simulink library "tpm"  (R2021b)
settings: Solver=VariableStepAuto  StartTime=0.0  StopTime=10.0  RelTol=1e-3
undefined symbols (not defined in the file or in its folder): ENUM_AN_LF, ENUM_AN_LR, ENUM_AN_RF, ENUM_AN_RR, ENUM_POWERSTA_OFF, ENUM_POWERSTA_OFFA, ENUM_POWERSTA_OFFC, ENUM_POWERSTA_ON, ENUM_POWERSTA_READY, ENUM_POWERSTA_STANDBY, ENUM_PWRSTASW_OFF, ENUM_PWRSTASW_OFFA, ENUM_PWRSTASW_OFFCHVCHRG, ENUM_PWRSTASW_STANDBY, ENUM_TPMSSNESORIDREGSTA_START, FALSE, KTPM_DataInVehSpdThreshold_kph, KTPM_Delay_raw8, KTPM_DiagLearn_flg, KTPM_TPMSModelVersion_raw, KTPM_WhlRotDir_enum_ovrdflg, KTPM_WhlRotDir_enum_ovrdval, TRUE, ZERO_FLOAT, ZERO_INT
libraries: simulink x58, $bdroot x27, hcu_lib x24
(part 7 of 9)

== system tpm/TPM/TPMS/TPMS/Learn/AutoLocation/IDIdentify/Subsystem7/Enabled Subsystem1 ==
  C : Inport
  LFM1 : Inport  Port=2
  Enable : EnablePort
  Data Type Conversion{1..8} (8 alike) : DataTypeConversion  OutDataTypeStr=int16
  Data Type Conversion9 : DataTypeConversion  OutDataTypeStr=uint8
  MATLAB Function : MATLAB Function  TreatAsAtomicUnit=on
  Unit Delay{1..8} (8 alike) : UnitDelay  SampleTime=-1  HasFrameUpgradeWarning=on
  S : Outport
  wires:
  [X9] -> MATLAB Function/10(X9)
  Unit Delay8/1 -> Data Type Conversion8/1
  Data Type Conversion8/1 -> [X9]
  MATLAB Function/9(Y9) -> Unit Delay8/1
  MATLAB Function/8(Y8) -> Unit Delay7/1
  Data Type Conversion7/1 -> [X8]
  Unit Delay7/1 -> Data Type Conversion7/1
  Unit Delay4/1 -> Data Type Conversion6/1
  MATLAB Function/7(Y7) -> Unit Delay4/1
  Data Type Conversion6/1 -> [X7]
  [X8] -> MATLAB Function/9(X8)
  [X7] -> MATLAB Function/8(X7)
  [X6] -> MATLAB Function/7(X6)
  [X5] -> MATLAB Function/6(X5)
  Data Type Conversion5/1 -> [X6]
  Data Type Conversion4/1 -> [X5]
  MATLAB Function/5(Y5) -> Unit Delay5/1
  MATLAB Function/6(Y6) -> Unit Delay6/1
  Unit Delay5/1 -> Data Type Conversion4/1
  Unit Delay6/1 -> Data Type Conversion5/1
  [X4] -> MATLAB Function/5(X4)
  [X3] -> MATLAB Function/4(X3)
  [X2] -> MATLAB Function/3(X2)
  Unit Delay3/1 -> Data Type Conversion3/1
  Unit Delay2/1 -> Data Type Conversion2/1
  Unit Delay1/1 -> Data Type Conversion1/1
  MATLAB Function/4(Y4) -> Unit Delay3/1
  MATLAB Function/3(Y3) -> Unit Delay2/1
  MATLAB Function/2(Y2) -> Unit Delay1/1
  C/1 -> MATLAB Function/1(C)
  MATLAB Function/1(S) -> Data Type Conversion9/1
  LFM1/1 -> MATLAB Function/2(Min)
  Data Type Conversion1/1 -> [X2]
  Data Type Conversion2/1 -> [X3]
  Data Type Conversion3/1 -> [X4]
  Data Type Conversion9/1 -> S/1

== system tpm/TPM/TPMS/TPMS/Learn/AutoLocation/IDIdentify/Subsystem7/Enabled Subsystem2 ==
  C : Inport
  LFM1 : Inport  Port=2
  Enable : EnablePort
  Data Type Conversion{1..8} (8 alike) : DataTypeConversion  OutDataTypeStr=int16
  Data Type Conversion9 : DataTypeConversion  OutDataTypeStr=uint8
  MATLAB Function : MATLAB Function  TreatAsAtomicUnit=on
  Unit Delay{1..8} (8 alike) : UnitDelay  SampleTime=-1  HasFrameUpgradeWarning=on
  S : Outport
  wires:
  Data Type Conversion3/1 -> [X4]
  Data Type Conversion2/1 -> [X3]
  Data Type Conversion1/1 -> [X2]
  LFM1/1 -> MATLAB Function/2(Min)
  MATLAB Function/1(S) -> Data Type Conversion9/1
  C/1 -> MATLAB Function/1(C)
  MATLAB Function/2(Y2) -> Unit Delay1/1
  MATLAB Function/3(Y3) -> Unit Delay2/1
  MATLAB Function/4(Y4) -> Unit Delay3/1
  Unit Delay1/1 -> Data Type Conversion1/1
  Unit Delay2/1 -> Data Type Conversion2/1
  Unit Delay3/1 -> Data Type Conversion3/1
  [X2] -> MATLAB Function/3(X2)
  [X3] -> MATLAB Function/4(X3)
  [X4] -> MATLAB Function/5(X4)
  Unit Delay6/1 -> Data Type Conversion5/1
  Unit Delay5/1 -> Data Type Conversion4/1
  MATLAB Function/6(Y6) -> Unit Delay6/1
  MATLAB Function/5(Y5) -> Unit Delay5/1
  Data Type Conversion4/1 -> [X5]
  Data Type Conversion5/1 -> [X6]
  [X5] -> MATLAB Function/6(X5)
  [X6] -> MATLAB Function/7(X6)
  [X7] -> MATLAB Function/8(X7)
  [X8] -> MATLAB Function/9(X8)
  Data Type Conversion6/1 -> [X7]
  MATLAB Function/7(Y7) -> Unit Delay4/1
  Unit Delay4/1 -> Data Type Conversion6/1
  Unit Delay7/1 -> Data Type Conversion7/1
  Data Type Conversion7/1 -> [X8]
  MATLAB Function/8(Y8) -> Unit Delay7/1
  MATLAB Function/9(Y9) -> Unit Delay8/1
  Data Type Conversion8/1 -> [X9]
  Unit Delay8/1 -> Data Type Conversion8/1
  [X9] -> MATLAB Function/10(X9)
  Data Type Conversion9/1 -> S/1

== system tpm/TPM/TPMS/TPMS/Learn/AutoLocation/IDIdentify/Subsystem7/Enabled Subsystem3 ==
  C : Inport
  LFM1 : Inport  Port=2
  Enable : EnablePort
  Data Type Conversion{1..8} (8 alike) : DataTypeConversion  OutDataTypeStr=int16
  Data Type Conversion9 : DataTypeConversion  OutDataTypeStr=uint8
  MATLAB Function : MATLAB Function  TreatAsAtomicUnit=on
  Unit Delay{1..8} (8 alike) : UnitDelay  SampleTime=-1  HasFrameUpgradeWarning=on
  S : Outport
  wires:
  [X9] -> MATLAB Function/10(X9)
  Unit Delay8/1 -> Data Type Conversion8/1
  Data Type Conversion8/1 -> [X9]
  MATLAB Function/9(Y9) -> Unit Delay8/1
  MATLAB Function/8(Y8) -> Unit Delay7/1
  Data Type Conversion7/1 -> [X8]
  Unit Delay7/1 -> Data Type Conversion7/1
  Unit Delay4/1 -> Data Type Conversion6/1
  MATLAB Function/7(Y7) -> Unit Delay4/1
  Data Type Conversion6/1 -> [X7]
  [X8] -> MATLAB Function/9(X8)
  [X7] -> MATLAB Function/8(X7)
  [X6] -> MATLAB Function/7(X6)
  [X5] -> MATLAB Function/6(X5)
  Data Type Conversion5/1 -> [X6]
  Data Type Conversion4/1 -> [X5]
  MATLAB Function/5(Y5) -> Unit Delay5/1
  MATLAB Function/6(Y6) -> Unit Delay6/1
  Unit Delay5/1 -> Data Type Conversion4/1
  Unit Delay6/1 -> Data Type Conversion5/1
  [X4] -> MATLAB Function/5(X4)
  [X3] -> MATLAB Function/4(X3)
  [X2] -> MATLAB Function/3(X2)
  Unit Delay3/1 -> Data Type Conversion3/1
  Unit Delay2/1 -> Data Type Conversion2/1
  Unit Delay1/1 -> Data Type Conversion1/1
  MATLAB Function/4(Y4) -> Unit Delay3/1
  MATLAB Function/3(Y3) -> Unit Delay2/1
  MATLAB Function/2(Y2) -> Unit Delay1/1
  C/1 -> MATLAB Function/1(C)
  MATLAB Function/1(S) -> Data Type Conversion9/1
  LFM1/1 -> MATLAB Function/2(Min)
  Data Type Conversion1/1 -> [X2]
  Data Type Conversion2/1 -> [X3]
  Data Type Conversion3/1 -> [X4]
  Data Type Conversion9/1 -> S/1

== system tpm/TPM/TPMS/TPMS/Learn/AutoLocation/IDIdentify/Subsystem7/Enabled Subsystem5 ==
  C : Inport
  LFM1 : Inport  Port=2
  Enable : EnablePort
  Data Type Conversion{1..8} (8 alike) : DataTypeConversion  OutDataTypeStr=int16
  Data Type Conversion9 : DataTypeConversion  OutDataTypeStr=uint8
  MATLAB Function : MATLAB Function  TreatAsAtomicUnit=on
  Unit Delay{1..8} (8 alike) : UnitDelay  SampleTime=-1  HasFrameUpgradeWarning=on
  S : Outport
  wires:
  Data Type Conversion3/1 -> [X4]
  Data Type Conversion2/1 -> [X3]
  Data Type Conversion1/1 -> [X2]
  LFM1/1 -> MATLAB Function/2(Min)
  MATLAB Function/1(S) -> Data Type Conversion9/1
  C/1 -> MATLAB Function/1(C)
  MATLAB Function/2(Y2) -> Unit Delay1/1
  MATLAB Function/3(Y3) -> Unit Delay2/1
  MATLAB Function/4(Y4) -> Unit Delay3/1
  Unit Delay1/1 -> Data Type Conversion1/1
  Unit Delay2/1 -> Data Type Conversion2/1
  Unit Delay3/1 -> Data Type Conversion3/1
  [X2] -> MATLAB Function/3(X2)
  [X3] -> MATLAB Function/4(X3)
  [X4] -> MATLAB Function/5(X4)
  Unit Delay6/1 -> Data Type Conversion5/1
  Unit Delay5/1 -> Data Type Conversion4/1
  MATLAB Function/6(Y6) -> Unit Delay6/1
  MATLAB Function/5(Y5) -> Unit Delay5/1
  Data Type Conversion4/1 -> [X5]
  Data Type Conversion5/1 -> [X6]
  [X5] -> MATLAB Function/6(X5)
  [X6] -> MATLAB Function/7(X6)
  [X7] -> MATLAB Function/8(X7)
  [X8] -> MATLAB Function/9(X8)
  Data Type Conversion6/1 -> [X7]
  MATLAB Function/7(Y7) -> Unit Delay4/1
  Unit Delay4/1 -> Data Type Conversion6/1
  Unit Delay7/1 -> Data Type Conversion7/1
  Data Type Conversion7/1 -> [X8]
  MATLAB Function/8(Y8) -> Unit Delay7/1
  MATLAB Function/9(Y9) -> Unit Delay8/1
  Data Type Conversion8/1 -> [X9]
  Unit Delay8/1 -> Data Type Conversion8/1
  [X9] -> MATLAB Function/10(X9)
  Data Type Conversion9/1 -> S/1

== system tpm/TPM/TPMS/TPMS/Learn/AutoLocation/WheelPosition/Subsystem/delay0 ==
  In1 : Inport
  Action Port : ActionPort
  Delay5 : Delay  DelayLength=0
  Out1 : Outport
  wires:
  In1/1 -> Delay5/1
  Delay5/1 -> Out1/1

== system tpm/TPM/TPMS/TPMS/Learn/AutoLocation/WheelPosition/Subsystem/delay1 ==
  In1 : Inport
  Action Port : ActionPort
  Delay5 : Delay  DelayLength=1
  Out1 : Outport
  wires:
  In1/1 -> Delay5/1
  Delay5/1 -> Out1/1

== system tpm/TPM/TPMS/TPMS/Learn/AutoLocation/WheelPosition/Subsystem/delay2 ==
  In1 : Inport
  Action Port : ActionPort
  Delay5 : Delay
  Out1 : Outport
  wires:
  In1/1 -> Delay5/1
  Delay5/1 -> Out1/1

== system tpm/TPM/TPMS/TPMS/Learn/AutoLocation/WheelPosition/Subsystem/delay3 ==
  In1 : Inport
  Action Port : ActionPort
  Delay5 : Delay  DelayLength=3
  Out1 : Outport
  wires:
  In1/1 -> Delay5/1
  Delay5/1 -> Out1/1

== system tpm/TPM/TPMS/TPMS/Learn/AutoLocation/WheelPosition/Subsystem/delay4 ==
  In1 : Inport
  Action Port : ActionPort
  Delay5 : Delay  DelayLength=4
  Out1 : Outport
  wires:
  Delay5/1 -> Out1/1
  In1/1 -> Delay5/1

== system tpm/TPM/TPMS/TPMS/Learn/AutoLocation/WheelPosition/Subsystem/delay5 ==
  In1 : Inport
  Action Port : ActionPort
  Delay5 : Delay  DelayLength=5
  Out1 : Outport
  wires:
  In1/1 -> Delay5/1
  Delay5/1 -> Out1/1

== system tpm/TPM/TPMS/TPMS/Learn/AutoLocation/WheelPosition/Subsystem/delay6 ==
  In1 : Inport
  Action Port : ActionPort
  Delay5 : Delay  DelayLength=6
  Out1 : Outport
  wires:
  Delay5/1 -> Out1/1
  In1/1 -> Delay5/1

== system tpm/TPM/TPMS/TPMS/Learn/AutoLocation/WheelPosition/Subsystem/delay7 ==
  In1 : Inport
  Action Port : ActionPort
  Delay5 : Delay  DelayLength=7
  Out1 : Outport
  wires:
  In1/1 -> Delay5/1
  Delay5/1 -> Out1/1

== system tpm/TPM/TPMS/TPMS/Learn/AutoLocation/WheelPosition/Subsystem/delay8 ==
  In1 : Inport
  Action Port : ActionPort
  Delay5 : Delay  DelayLength=8
  Out1 : Outport
  wires:
  Delay5/1 -> Out1/1
  In1/1 -> Delay5/1

== matlab function tpm/TPM/TPMS/TPMS/Learn/AutoLocation/IDIdentify/Subsystem7/Enabled Subsystem5/MATLAB Function ==
  data: C input; S output; Min input; X2 input; X3 input; X4 input; Y2 output; Y3 output; Y4 output; X5 input; X6 input; X7 input; X8 input; X9 input; Y5 output; Y6 output; Y7 output; Y8 output; Y9 output
function [S,Y2,Y3,Y4,Y5,Y6,Y7,Y8,Y9]   = fcn(C,Min,X2,X3,X4,X5,X6,X7,X8,X9)
Y=int16([X2 X3 X4 X5 X6 X7 X8 X9 Min]);
if (C<9)
    S=300;
else
    B=sort(Y);
    D=zeros(1,length(B));
    for i=1:1:length(D)
        if (i~=length(D))
            D(i)=B(i+1)-B(i);
        else
            if (B(length(D))-B(1)>B(1)+96-B(length(D)))
                D(length(D))=B(1)+96-B(length(D));
            else
                D(length(D))=B(length(D))-B(1);
            end
        end
    end

    [K,I]=sort(D);
    S=sum(K(1:7));
end
Y2=Y(2);
Y3=Y(3);
Y4=Y(4);
Y5=Y(5);
Y6=Y(6);
Y7=Y(7);
Y8=Y(8);
Y9=Y(9);

== stateflow chart tpm/TPM/TPMS/TPMS/Learn/AutoLocation/WheelPosition/Chart2 ==
  state Start
    state Forward
      en:
      a=(VTPM_RFWpos_raw+Delta);
      b=(VTPM_RFWpos_raw+Delta)/96;
      VTPM_RFWpos_raw=a-b*96;
    state Else
    state Backward
      en:
      a=(VTPM_RFWpos_raw+Delta);
      b=(VTPM_RFWpos_raw+Delta)/96;
      VTPM_RFWpos_raw=a-b*96;
    (default) -> (junction 54) : {VTPM_RFWpos_raw=0; Delta=0; PulseCountBuf=VINP_RFPulseCount_cnt;}
    Start -> (junction 54) : [hasChanged(VINP_RFPulseCount_cnt)]....
        | {Delta=VINP_RFPulseCount_cnt-PulseCountBuf;
        | PulseCountBuf=VINP_RFPulseCount_cnt;}
    (junction 54) -> (junction 47) [order 1] : [VPMM_PowerSta_enum!=ENUM_PWRSTASW_OFF&&....
        |  VPMM_PowerSta_enum!=ENUM_PWRSTASW_OFFCHVCHRG&&...
        |  VPMM_PowerSta_enum!=ENUM_PWRSTASW_OFFA&&....
        |  VPMM_PowerSta_enum!=ENUM_PWRSTASW_STANDBY&&....
        |  VINP_RFPulseCountV_flg==false]
    (junction 47) -> (junction 6) [order 1] : [VTPM_RFWhlRotDir_enum==1]
    (junction 6) -> Forward [order 1] : [Delta>0]
    (junction 54) -> Else [order 2]
    (junction 47) -> (junction 48) [order 2]
    (junction 6) -> (junction 10) [order 2] : [Delta<0]
    (junction 10) -> Forward : {Delta=Delta+256;}
    (junction 48) -> Else [order 2]
    (junction 48) -> (junction 14) [order 1] : [VTPM_RFWhlRotDir_enum==2]
    (junction 14) -> Backward [order 1] : [Delta>0]{Delta=-Delta+96;}
    (junction 14) -> (junction 16) [order 2] : [Delta<0]
    (junction 16) -> Backward : {Delta=-Delta+128;}
  data: VPMM_PowerSta_enum input; VINP_RFPulseCount_cnt input; VINP_RFPulseCountV_flg input; VTPM_RFWhlRotDir_enum input; VTPM_RFWpos_raw output int16; a local int16; b local int16; Delta local int16; PulseCountBuf local int16; ENUM_PWRSTASW_OFF parameter; ENUM_PWRSTASW_OFFA parameter; ENUM_PWRSTASW_OFFCHVCHRG parameter; ENUM_PWRSTASW_STANDBY parameter

== stateflow chart tpm/TPM/TPMS/TPMS/Learn/AutoLocation/IDIdentify/unlearnsensorfail /Chart ==
  state FLSAH
    en:
    VTPM_unlearnSfali_flg=VINP_FlashunlearnSfali_flg;
  state VINP_TPMSResButt_flg
    en:
    VTPM_unlearnSfali_flg=false;
    VTPM_GSX_flg=false;
    VTPM_Idunlock_cnt=0;
    VTPM_GSS1_cnt=0;
    VTPM_GSS2_cnt=0;
    VTPM_GSS3_cnt=0;
    VTPM_GSS4_cnt=0;
    VTPM_Idunlockkeep_cnt=0;
    VTPM_unlockpopup_flg=false;
  state ALfin
    en:
    VTPM_GSX_flg=false;
    VTPM_unlearnSfali_flg=false;
    VTPM_unlockpopup_flg=false;
  state vehspeedthreshold
    en:
    VTPM_Idunlock_cnt=0;
    VTPM_GSS1_cnt=0;
    VTPM_GSS2_cnt=0;
    VTPM_GSS3_cnt=0;
    VTPM_GSS4_cnt=0;
  state locationdone
    en:
    VTPM_GSX_flg=false;
    VTPM_unlearnSfali_flg=false;
    VTPM_unlockpopup_flg=false;
  state unlearnsensorfail
    (default) -> (junction 83) : {VTPM_Idunlock_cnt=0;
        | VTPM_GSS1_cnt=0;
        | VTPM_GSS2_cnt=0;
        | VTPM_GSS3_cnt=0;
        | VTPM_GSS4_cnt=0;
        | }
    unlearnsensorfail -> (junction 83) [order 1] : [!VTPM_IDLOCK_flg]
    (junction 83) -> (junction 86) [order 1] : [VTPM_IDLOCK_flg]
    (junction 83) -> (junction 211) [order 2] : {VTPM_Idunlock_cnt+=1;
        | VTPM_Idunlockkeep_cnt+=1;}
    (junction 86) -> (junction 90) : {VTPM_unlockpopup_flg=false;}
    (junction 211) -> (junction 212) [order 1] : [VTPM_Idunlockkeep_cnt==30000||VTPM_unlockpopup_flg==true]
    (junction 211) -> (junction 215) [order 2]
    (junction 212) -> (junction 88) : {VTPM_unlockpopup_flg=true;}
    (junction 88) -> (junction 103) [order 1] : [VTPM_Idunlock_cnt==48000||VTPM_unlearnSfali_flg==true]
    (junction 88) -> (junction 105) [order 2]
    (junction 103) -> (junction 107) : {VTPM_unlearnSfali_flg=true;}
    unlearnsensorfail -> (junction 90) [order 2] : [VTPM_GSX_flg==true||VTPM_IDLOCK_flg]{VTPM_unlockpopup_flg=false;}
    (junction 90) -> (junction 132) [order 1] : [VTPM_GS1_flg==true]
    (junction 90) -> (junction 144) [order 2]
    (junction 132) -> (junction 150) : {
        | VTPM_GSS2_cnt+=1;
        | VTPM_GSS3_cnt+=1;
        | VTPM_GSS4_cnt+=1;
        | VTPM_GSS1_cnt=0;
        | }
    (junction 144) -> (junction 152) [order 1] : [VTPM_GS2_flg==true]
    (junction 144) -> (junction 156) [order 2]
    (junction 152) -> (junction 154) : {
        | VTPM_GSS1_cnt+=1;
        | VTPM_GSS3_cnt+=1;
        | VTPM_GSS4_cnt+=1;
        | VTPM_GSS2_cnt=0;
        | }
    (junction 156) -> (junction 158) [order 1] : [VTPM_GS3_flg==true]
    (junction 156) -> (junction 162) [order 2]
    (junction 158) -> (junction 160) : {VTPM_GSS1_cnt+=1;
        | VTPM_GSS2_cnt+=1;
        | VTPM_GSS4_cnt+=1;
        | VTPM_GSS3_cnt=0;
        | }
    (junction 162) -> (junction 168) [order 1] : [VTPM_GS4_flg==true]
    (junction 162) -> (junction 172) [order 2] : {
        | VTPM_GSS1_cnt+=1;
        | VTPM_GSS2_cnt+=1;
        | VTPM_GSS3_cnt+=1;
        | VTPM_GSS4_cnt+=1;
        | }
    (junction 168) -> (junction 170) : {
        | VTPM_GSS1_cnt+=1;
        | VTPM_GSS2_cnt+=1;
        | VTPM_GSS3_cnt+=1;
        | VTPM_GSS4_cnt=0;
        | }
    (junction 170) -> (junction 172)
    (junction 160) -> (junction 170)
    (junction 154) -> (junction 160)
    (junction 150) -> (junction 154)
    (junction 172) -> (junction 179) : {
        | VTPM_GSX_flg=true;
        | }
    (junction 179) -> (junction 176) [order 1] : [VTPM_GSS1_cnt==18000||VTPM_GSS2_cnt==18000||VTPM_GSS3_cnt==18000||VTPM_GSS4_cnt==18000]
    (junction 179) -> (junction 191) [order 2]
    (junction 176) -> (junction 181) : {VTPM_unlearnSfali_flg=true;
        | VTPM_GSX_flg=false;
        | }
  (default) -> FLSAH
  FLSAH -> unlearnsensorfail [order 3]
  FLSAH -> ALfin [order 2] : [VTPM_ALLFIN_flg]
  FLSAH -> locationdone [order 1] : [VINP_ChkStorge_flg||VINP_TPMSStorge_flg||VTPM_TPMSmanualDone_flg]
  ALfin -> (junction 257) [order 1] : [VINP_TPMSResButt_flg]
  (junction 257) -> VINP_TPMSResButt_flg
  locationdone -> (junction 257) [order 1] : [VINP_TPMSResButt_flg]
  unlearnsensorfail -> ALfin [order 3] : [VTPM_ALLFIN_flg]
  ALfin -> unlearnsensorfail [order 2] : [!VTPM_ALLFIN_flg]
  vehspeedthreshold -> VINP_TPMSResButt_flg [order 1] : [VINP_TPMSResButt_flg]
  unlearnsensorfail -> locationdone [order 2] : [VINP_ChkStorge_flg||VINP_TPMSStorge_flg||VTPM_TPMSmanualDone_flg]
  locationdone -> unlearnsensorfail [order 2] : [!VINP_ChkStorge_flg&&!VINP_TPMSStorge_flg&&....
      | !VTPM_TPMSmanualDone_flg]
  unlearnsensorfail -> VINP_TPMSResButt_flg [order 1] : [VINP_TPMSResButt_flg]
  VINP_TPMSResButt_flg -> unlearnsensorfail
  vehspeedthreshold -> unlearnsensorfail [order 2] : [VINP_VehSpeed_kph>=25]
  unlearnsensorfail -> vehspeedthreshold [order 4] : [VINP_VehSpeed_kph<25]
  data: VTPM_ALLFIN_flg input; VINP_VehSpeed_kph input; VTPM_IDLOCK_flg input; VTPM_Idunlock_cnt local uint32; VTPM_GS2_flg input; VTPM_GS3_flg input; VTPM_GS4_flg input; VTPM_GS1_flg input; VTPM_unlearnSfali_flg output boolean; VTPM_GSX_flg local boolean; VINP_TPMSResButt_flg input; VINP_FlashunlearnSfali_flg input; VINP_ChkStorge_flg input; VINP_TPMSStorge_flg input; VTPM_GSS1_cnt local uint32; VTPM_GSS2_cnt local uint32; VTPM_GSS3_cnt local uint32; VTPM_GSS4_cnt local uint32; VTPM_unlockpopup_flg output boolean; VTPM_Idunlockkeep_cnt local uint16; VTPM_TPMSmanualDone_flg input boolean

== stateflow chart tpm/TPM/TPMS/TPMS/Learn/AutoLocation/IDIdentify/Subsystem2/Chart ==
  state Sample [parallel]
    settings: executionOrder=1
    state DataNotEnough
    state Regisiter
      en:
      C=C+1;
      LFM=LF_PC;
      RFM=RF_PC;
      LRM=LR_PC;
      RRM=RR_PC;
    (default) -> DataNotEnough : {C=0;}
    Regisiter -> (junction 513) [order 2] : [GS]
    DataNotEnough -> Regisiter [order 2] : [!VINP_TPMSResButt_flg&&GS]
    (junction 513) -> (junction 514)
    (junction 514) -> Regisiter
    Regisiter -> DataNotEnough [order 1] : [VINP_TPMSResButt_flg]{C=0;}
    Regisiter -> (junction 528) [order 3] : [VPMM_PowerSta_enum!=ENUM_POWERSTA_ON&&...
        | VPMM_PowerSta_enum!=ENUM_POWERSTA_READY
        | ]
    (junction 528) -> (junction 532) : {C=0;}
    (junction 532) -> DataNotEnough
    DataNotEnough -> DataNotEnough [order 1] : [VINP_TPMSResButt_flg]{C=0;}
  data: VINP_TPMSResButt_flg input; VPMM_PowerSta_enum input; GS input; LR_PC input; LF_PC input; RR_PC input; RF_PC input; LFM output int16; LRM output int16; RRM output int16; RFM output int16; C output uint8; ENUM_POWERSTA_READY parameter; ENUM_POWERSTA_ON parameter

== stateflow chart tpm/TPM/TPMS/TPMS/Send/Alarm/Chart ==
  settings: sampleTime=StepSize
  state LF_PDectect [parallel]
    settings: executionOrder=4
    state OFF
      en:LFPressIndi=0;
    state Detect
      state NoWarning
        en:LFPressIndi=0;
      state LowPressure
        en:
        LFPressIndi=2;
      LF_PDectect.Detect.NoWarning -> LF_PDectect.Detect.LowPressure : [(LFPindi==1||LFPindi==2||LFPindi==3)&&LFP20<LFPalarm]
      LF_PDectect.Detect.LowPressure -> LF_PDectect.Detect.NoWarning : [LFPindi==0||LFP20>=LFPalarm+8.14]
    (default) -> LF_PDectect.OFF
    LF_PDectect.OFF -> LF_PDectect.Detect.NoWarning : [PwrSta>3]
    LF_PDectect.Detect -> LF_PDectect.OFF : [PwrSta<=3]
  state LR_PDectect [parallel]
    settings: executionOrder=6
    state OFF
      en:LRPressIndi=0;
    state Detect
      state NoWarning
        en:LRPressIndi=0;
      state LowPressure
        en:
        LRPressIndi=2;
      LR_PDectect.Detect.NoWarning -> LR_PDectect.Detect.LowPressure : [(LRPindi==1||LRPindi==2||LRPindi==3)&&LRP20<LRPalarm]
      LR_PDectect.Detect.LowPressure -> LR_PDectect.Detect.NoWarning : [LRPindi==0||LRP20>=LRPalarm+8.14]
    (default) -> LR_PDectect.OFF
    LR_PDectect.OFF -> LR_PDectect.Detect.NoWarning : [PwrSta>3]
    LR_PDectect.Detect -> LR_PDectect.OFF : [PwrSta<=3]
  state RF_PDectect [parallel]
    settings: executionOrder=5
    state OFF
      en:RFPressIndi=0;
    state Detect
      state NoWarning
        en:RFPressIndi=0;
      state LowPressure
        en:
        RFPressIndi=2;
      RF_PDectect.Detect.NoWarning -> RF_PDectect.Detect.LowPressure : [(RFPindi==1||RFPindi==2||RFPindi==3)&&RFP20<RFPalarm]
      RF_PDectect.Detect.LowPressure -> RF_PDectect.Detect.NoWarning : [RFPindi==0||RFP20>=RFPalarm+8.14]
    (default) -> RF_PDectect.OFF
    RF_PDectect.OFF -> RF_PDectect.Detect.NoWarning : [PwrSta>3]
    RF_PDectect.Detect -> RF_PDectect.OFF : [PwrSta<=3]
  state RR_PDectect [parallel]
    settings: executionOrder=7
    state OFF
      en:RRPressIndi=0;
    state Detect
      state NoWarning
        en:RRPressIndi=0;
      state LowPressure
        en:
        RRPressIndi=2;
      RR_PDectect.Detect.NoWarning -> RR_PDectect.Detect.LowPressure : [(RRPindi==1||RRPindi==2||RRPindi==3)&&RRP20<RRPalarm]
      RR_PDectect.Detect.LowPressure -> RR_PDectect.Detect.NoWarning : [RRPindi==0||RRP20>=RRPalarm+8.14]
    (default) -> RR_PDectect.OFF
    RR_PDectect.OFF -> RR_PDectect.Detect.NoWarning : [PwrSta>3]
    RR_PDectect.Detect -> RR_PDectect.OFF : [PwrSta<=3]
  state TPMSWarnIND [parallel]
    settings: executionOrder=3
    state OFF
      en:TPMSWarnIndi=0;
    state Process
      state Standby
        state Unlearn
          en:
          TPMSWarnIndi=3;
        state learn
          en:
          TPMSWarnIndi=0;
        (default) -> (junction 1978)
        (junction 1978) -> Unlearn [order 2]
        (junction 1978) -> learn [order 1] : [VTPM_Done_flg]
        Unlearn -> learn : [VTPM_Done_flg]
        learn -> Unlearn : [!VTPM_Done_flg]
      state LowP
        en:TPMSWarnIndi=1;
      state CANFail
      state FailAlarm
        state SystemFail
          en:TPMSWarnIndi=2;
        state SystemFail2
          en:TPMSWarnIndi=1;
        (default) -> SystemFail
        SystemFail -> SystemFail2 : [after(6000,tick)]
      (default) -> Standby
      Standby -> LowP [order 1] : [LFPressIndi==2||RFPressIndi==2||LRPressIndi==2||RRPressIndi==2]
      (junction 1946) -> Standby : [LFPressIndi==0&&RFPressIndi==0&&LRPressIndi==0&&RRPressIndi==0]
      LowP -> (junction 1946) [order 1]
      FailAlarm -> (junction 1946) : [!SF&&!VTPM_unlearnSfali_flg]
      LowP -> FailAlarm [order 2] : [SF||VTPM_unlearnSfali_flg]
      Standby -> CANFail [order 3] : [!CANValid]
      Standby -> FailAlarm [order 2] : [SF||VTPM_unlearnSfali_flg]
      CANFail -> FailAlarm : [after(250,tick)]
    (default) -> TPMSWarnIND.OFF
    TPMSWarnIND.OFF -> Process : [PwrSta>3]
    Process -> TPMSWarnIND.OFF : [PwrSta<=3]
  state CailbrationTip [parallel]
    settings: executionOrder=1
    state OFF
      en:CWheelTips=0;
    state ON
      state Fail
        en:CWheelTips=2;
      state StandBy
        en:CWheelTips=0;
      state ButtClick
        en:CWheelTips=0;
      state Success
        en:CWheelTips=1;
      (junction 1893) -> (junction 1896) [order 1]
      (junction 1896) -> Fail : [LFPindi==2||RFPindi==2||LRPindi==2||RRPindi==2]
      (junction 1893) -> CailbrationTip.ON.StandBy [order 2]
      CailbrationTip.ON.ButtClick -> (junction 1896) [order 1]
      Fail -> CailbrationTip.ON.ButtClick : [LFPindi!=2&&RFPindi!=2&&LRPindi!=2&&RRPindi!=2]
      CailbrationTip.ON.StandBy -> CailbrationTip.ON.ButtClick : [TireCailButt||ResetButt]
      CailbrationTip.ON.ButtClick -> CailbrationTip.ON.Success [order 2] : [VTPM_IDLOCK_flg&&LFPindi==1&&RFPindi==1&&LRPindi==1&&RRPindi==1]
      CailbrationTip.ON.Success -> CailbrationTip.ON.StandBy : [after (500,tick)]
    (default) -> CailbrationTip.OFF
    CailbrationTip.ON -> CailbrationTip.OFF : [PwrSta<=3]
    CailbrationTip.OFF -> (junction 1893) : [PwrSta>3]
  state AutoLocationTip [parallel]
    settings: executionOrder=2
    state OFF
      en:AutoLTips=3;
    state ON
      state Popup
        en:AutoLTips=2;
      state StandBy
        en:AutoLTips=0;
      state ButtClick
        en:AutoLTips=0;
      state Success
        en:AutoLTips=1;
      AutoLocationTip.ON.StandBy -> Popup [order 1] : [VTPM_unlockpopup_flg]
      Popup -> AutoLocationTip.ON.ButtClick [order 1] : [ResetButt]
      AutoLocationTip.ON.ButtClick -> Popup [order 1] : [VTPM_unlockpopup_flg]
      Popup -> AutoLocationTip.ON.Success [order 2] : [VTPM_Done_flg]
      AutoLocationTip.ON.StandBy -> AutoLocationTip.ON.ButtClick [order 2] : [ResetButt]
      AutoLocationTip.ON.ButtClick -> AutoLocationTip.ON.Success [order 2] : [VTPM_Done_flg]
      AutoLocationTip.ON.Success -> AutoLocationTip.ON.StandBy : [after(500,tick)]
    (default) -> AutoLocationTip.OFF
    AutoLocationTip.OFF -> AutoLocationTip.ON.StandBy : [PwrSta>3]
    AutoLocationTip.ON -> AutoLocationTip.OFF : [PwrSta<=3]
  data: PwrSta input; LFPressIndi output uint8; RFPressIndi output uint8; LRPressIndi output uint8; RRPressIndi output uint8; TPMSWarnIndi output uint8; SF input; VTPM_Done_flg input; LFPindi input; RFPindi input; RRPindi input; LRPindi input; LFP20 input; LRP20 input; RFP20 input; RRP20 input; LFPalarm input; RFPalarm input; LRPalarm input; RRPalarm input; CWheelTips output uint8; AutoLTips output uint8; TireCailButt input; ResetButt input; CANValid input; VTPM_unlearnSfali_flg input boolean; VTPM_unlockpopup_flg input boolean; VTPM_IDLOCK_flg input

== stateflow chart tpm/TPM/TPMS/TPMS/Send/ResetAllow&CalibrateAllow/Chart ==
  state GearSta [parallel]
    settings: executionOrder=1
    state PGear
      en:
      FATallow=true;
    state StandBy
      en:
      FATallow=false;
    (default) -> GearSta.StandBy
    GearSta.StandBy -> PGear : [VTQD_GearActualPosn_enum == ENUM_GEARACTUALPOSN_P]
    PGear -> GearSta.StandBy : [VTQD_GearActualPosn_enum != ENUM_GEARACTUALPOSN_P]
  state ResetBtnSta [parallel]
    settings: executionOrder=2
    state StandBy
      en:
      VTPM_TPMSResButtAllow_flg=false;
    state Allow
      en:
      VTPM_TPMSResButtAllow_flg=true;
    (default) -> ResetBtnSta.StandBy
    ResetBtnSta.StandBy -> ResetBtnSta.Allow : [VINP_VehSpeed_kph<KTPM_DataInVehSpdThreshold_kph&&FATallow&&!VINP_TPMSResButt_flg]
    ResetBtnSta.Allow -> ResetBtnSta.StandBy : [VINP_VehSpeed_kph>=KTPM_DataInVehSpdThreshold_kph||!FATallow||VINP_TPMSResButt_flg]
  state CalibrateBtnSta [parallel]
    settings: executionOrder=3
    state StandBy
      en:
      VTPM_TPMSCaliButtAllow_flg=false;
    state fivesec
    state Allow
      en:
      VTPM_TPMSCaliButtAllow_flg=true;
    (default) -> CalibrateBtnSta.StandBy
    CalibrateBtnSta.StandBy -> fivesec : [!VINP_TPMSResButt_flg&&!VINP_TPMSCaliButt_flg&&VTPM_Done_flg]
    fivesec -> CalibrateBtnSta.Allow : [after(500,tick)&&VINP_VehSpeed_kph<=eps]
    CalibrateBtnSta.Allow -> CalibrateBtnSta.StandBy : [VINP_TPMSResButt_flg||VINP_TPMSCaliButt_flg||!VTPM_Done_flg||VINP_VehSpeed_kph>0]
  data: VTQD_GearActualPosn_enum input; VINP_VehSpeed_kph input; VINP_TPMSResButt_flg input; VINP_TPMSCaliButt_flg input; VTPM_TPMSCaliButtAllow_flg output boolean; VTPM_TPMSResButtAllow_flg output boolean; VTPM_Done_flg input; FATallow local boolean; ENUM_GEARACTUALPOSN_P parameter; eps local double; KTPM_DataInVehSpdThreshold_kph input single

== stateflow chart tpm/TPM/TPMS/TPMS/Send/DATA/RFSW ==
  state OFF
  state ON
    state StandBy
    state Reset_Cail
      en:
      VTPM_RFWheelTemp_C=215;
    state Received
      en:VTPM_RFWheelPress_raw8=VINP_Pin_raw8;
      VTPM_RFWheelTemp_C=VTPM_Tin_c;
      VTPM_RFBatWarn_flg=VINP_BatteryLow_flg;
      VTPM_RFP20_raw8=uint8(((double(VTPM_RFWheelPress_raw8)*1.72+151)*(273+20)/(273+double(VTPM_RFWheelTemp_C))-151)/1.72);
      VTPM_RFWheelDebug_flg=true;
      VTPM_RFSensorMode_flg=VINP_FAT_flg;
      VTPM_RFSensorFail_flg=false;
      ex:
      VTPM_RFWheelDebug_flg=false;
      VTPM_RFSensorMode_flg=false;
    state PreSenfail
    state SensorFail
      en:VTPM_RFSensorFail_flg=true;
    (default) -> StandBy
    StandBy -> Reset_Cail [order 1] : [VINP_TPMSResButt_flg]
    Reset_Cail -> StandBy
    StandBy -> Received [order 2] : [VTPM_RFSW_flg==true]
    Received -> StandBy : [VTPM_RFSW_flg==false]
    SensorFail -> StandBy [order 2] : [!VTPM_Done_flg]
        | {VTPM_RFSensorFail_flg=false;
        | }
    PreSenfail -> StandBy [order 2] : [VINP_VehSpeed_kph<25||!VTPM_Done_flg]
    StandBy -> PreSenfail [order 3] : [VINP_VehSpeed_kph>=25&&VTPM_Done_flg]
    PreSenfail -> Received [order 1] : [VTPM_RFSW_flg==true]
    SensorFail -> Received [order 1] : [VTPM_RFSW_flg==true]
    PreSenfail -> SensorFail [order 3] : [after(48000,tick)]
  (default) -> OFF
  ON -> OFF : [VPMM_PowerSta_enum==ENUM_POWERSTA_OFF||...
      | VPMM_PowerSta_enum==ENUM_POWERSTA_OFFC||...
      | VPMM_PowerSta_enum==ENUM_POWERSTA_OFFA||...
      | VPMM_PowerSta_enum==ENUM_POWERSTA_STANDBY
      | ]
  OFF -> ON : [VPMM_PowerSta_enum==ENUM_POWERSTA_ON||...
      | VPMM_PowerSta_enum==ENUM_POWERSTA_READY]
  data: VTPM_RFSW_flg input; VINP_Pin_raw8 input; VTPM_Tin_c input; VINP_BatteryLow_flg input; VTPM_RFWheelPress_raw8 output uint8; VTPM_RFWheelTemp_C output single; VTPM_RFBatWarn_flg output boolean; VTPM_RFSensorFail_flg output boolean; VPMM_PowerSta_enum input; VTPM_RFP20_raw8 output uint8; VINP_FAT_flg input; VTPM_RFWheelDebug_flg output boolean; VTPM_RFSensorMode_flg output boolean; ENUM_POWERSTA_ON parameter; ENUM_POWERSTA_READY parameter; VINP_VehSpeed_kph input; VTPM_Done_flg input; ENUM_POWERSTA_OFF parameter; ENUM_POWERSTA_OFFA parameter; ENUM_POWERSTA_OFFC parameter; ENUM_POWERSTA_STANDBY parameter; VINP_TPMSResButt_flg input

== stateflow chart tpm/TPM/TPMS/TPMS/Send/DATA/LRSW ==
  state OFF
  state ON
    state Reset_Cail
      en:
      VTPM_LRWheelTemp_C=215;
    state StandBy
    state Received
      en:VTPM_LRWheelPress_raw8=VINP_Pin_raw8;
      VTPM_LRWheelTemp_C=VTPM_Tin_c;
      VTPM_LRBatWarn_flg=VINP_BatteryLow_flg;
      VTPM_LRP20_raw8=uint8(((double(VTPM_LRWheelPress_raw8)*1.72+151)*(273+20)/(273+double(VTPM_LRWheelTemp_C))-151)/1.72);
      VTPM_LRWheelDebug_flg=true;
      VTPM_LRSensorMode_flg=VINP_FAT_flg;
      VTPM_LRSensorFail_flg=false;
      ex:
      VTPM_LRWheelDebug_flg=false;
      VTPM_LRSensorMode_flg=false;
    state PreSenfail
    state SensorFail
      en:VTPM_LRSensorFail_flg=true;
    (default) -> StandBy
    StandBy -> Reset_Cail [order 1] : [VINP_TPMSResButt_flg]
    Reset_Cail -> StandBy
    StandBy -> Received [order 2] : [VTPM_LRSW_flg==true]
    Received -> StandBy : [VTPM_LRSW_flg==false]
    SensorFail -> StandBy [order 2] : [!VTPM_Done_flg]
        | {VTPM_LRSensorFail_flg=false;
        | }
    PreSenfail -> StandBy [order 2] : [VINP_VehSpeed_kph<25||!VTPM_Done_flg]
    StandBy -> PreSenfail [order 3] : [VINP_VehSpeed_kph>=25&&VTPM_Done_flg]
    PreSenfail -> Received [order 1] : [VTPM_LRSW_flg==true]
    SensorFail -> Received [order 1] : [VTPM_LRSW_flg==true]
    PreSenfail -> SensorFail [order 3] : [after(48000,tick)]
  (default) -> OFF
  ON -> OFF : [VPMM_PowerSta_enum==ENUM_POWERSTA_OFF||...
      | VPMM_PowerSta_enum==ENUM_POWERSTA_OFFC||...
      | VPMM_PowerSta_enum==ENUM_POWERSTA_OFFA||...
      | VPMM_PowerSta_enum==ENUM_POWERSTA_STANDBY
      | ]
  OFF -> ON : [VPMM_PowerSta_enum==ENUM_POWERSTA_ON||...
      | VPMM_PowerSta_enum==ENUM_POWERSTA_READY]
  data: VTPM_LRSW_flg input; VINP_Pin_raw8 input; VTPM_Tin_c input; VINP_BatteryLow_flg input; VTPM_LRWheelPress_raw8 output uint8; VTPM_LRWheelTemp_C output single; VTPM_LRBatWarn_flg output boolean; VTPM_LRSensorFail_flg output boolean; VPMM_PowerSta_enum input; VTPM_LRP20_raw8 output uint8; VINP_FAT_flg input; VTPM_LRWheelDebug_flg output boolean; VTPM_LRSensorMode_flg output boolean; ENUM_POWERSTA_ON parameter; ENUM_POWERSTA_READY parameter; VINP_VehSpeed_kph input; VTPM_Done_flg input; ENUM_POWERSTA_OFF parameter; ENUM_POWERSTA_OFFA parameter; ENUM_POWERSTA_OFFC parameter; ENUM_POWERSTA_STANDBY parameter; VINP_TPMSResButt_flg input

== stateflow chart tpm/TPM/TPMS/TPMS/Send/DATA/RRSW ==
  state OFF
  state ON
    state Reset_Cail
      en:
      VTPM_RRWheelTemp_C=215;
    state StandBy
    state Received
      en:VTPM_RRWheelPress_raw8=VINP_Pin_raw8;
      VTPM_RRWheelTemp_C=VTPM_Tin_c;
      VTPM_RRBatWarn_flg=VINP_BatteryLow_flg;
      VTPM_RRP20_raw8=uint8(((double(VTPM_RRWheelPress_raw8)*1.72+151)*(273+20)/(273+double(VTPM_RRWheelTemp_C))-151)/1.72);
      VTPM_RRWheelDebug_flg=true;
      VTPM_RRSensorMode_flg=VINP_FAT_flg;
      VTPM_RRSensorFail_flg=false;
      ex:
      VTPM_RRWheelDebug_flg=false;
      VTPM_RRSensorMode_flg=false;
    state PreSenfail
    state SensorFail
      en:VTPM_RRSensorFail_flg=true;
    (default) -> StandBy
    StandBy -> Reset_Cail [order 2] : [VINP_TPMSResButt_flg]
    Reset_Cail -> StandBy
    StandBy -> Received [order 1] : [VTPM_RRSW_flg==true]
    Received -> StandBy : [VTPM_RRSW_flg==false]
    SensorFail -> StandBy [order 2] : [!VTPM_Done_flg]
        | {VTPM_RRSensorFail_flg=false;
        | }
    PreSenfail -> StandBy [order 2] : [VINP_VehSpeed_kph<25||!VTPM_Done_flg]
    StandBy -> PreSenfail [order 3] : [VINP_VehSpeed_kph>=25&&VTPM_Done_flg]
    PreSenfail -> Received [order 1] : [VTPM_RRSW_flg==true]
    SensorFail -> Received [order 1] : [VTPM_RRSW_flg==true]
    PreSenfail -> SensorFail [order 3] : [after(48000,tick)]
  (default) -> OFF
  ON -> OFF : [VPMM_PowerSta_enum==ENUM_POWERSTA_OFF||...
      | VPMM_PowerSta_enum==ENUM_POWERSTA_OFFC||...
      | VPMM_PowerSta_enum==ENUM_POWERSTA_OFFA||...
      | VPMM_PowerSta_enum==ENUM_POWERSTA_STANDBY
      | ]
  OFF -> ON : [VPMM_PowerSta_enum==ENUM_POWERSTA_ON||...
      | VPMM_PowerSta_enum==ENUM_POWERSTA_READY]
  data: VTPM_RRSW_flg input; VINP_Pin_raw8 input; VTPM_Tin_c input; VINP_BatteryLow_flg input; VTPM_RRWheelPress_raw8 output uint8; VTPM_RRWheelTemp_C output single; VTPM_RRBatWarn_flg output boolean; VTPM_RRSensorFail_flg output boolean; VPMM_PowerSta_enum input; VTPM_RRP20_raw8 output uint8; VINP_FAT_flg input; VTPM_RRWheelDebug_flg output boolean; VTPM_RRSensorMode_flg output boolean; ENUM_POWERSTA_ON parameter; ENUM_POWERSTA_READY parameter; VINP_VehSpeed_kph input; VTPM_Done_flg input; ENUM_POWERSTA_OFF parameter; ENUM_POWERSTA_OFFA parameter; ENUM_POWERSTA_OFFC parameter; ENUM_POWERSTA_STANDBY parameter; VINP_TPMSResButt_flg input

== stateflow chart tpm/TPM/TPMS/TPMS/Learn/AutoLocation/Subsystem1/Chart ==
  state StandBy
    en:TPMSTLCmd=0;
    fDone=0;
  state Learning
    en:TPMSTLCmd=1;
    LProgress=2;
    state WaitDatain
    (default) -> WaitDatain
    WaitDatain -> (junction 6) : [DataIn&&VINP_TPMSTrigger_flg]
    (junction 6) -> (junction 61) [order 1] : [VTPM_WritingCnt_enum==0]
        | {ID1=IDin;....
        | ID1pressure=VINP_Pin_raw8;....
        | ID1Temp=VINP_Tin_raw8;}
    (junction 6) -> (junction 33) [order 2] : [ID1!=IDin]
    (junction 61) -> (junction 63)
    (junction 33) -> (junction 63) [order 1] : [VTPM_WritingCnt_enum==1]
        | {ID2=IDin;....
        | ID2pressure=VINP_Pin_raw8;....
        | ID2Temp=VINP_Tin_raw8;}
    (junction 33) -> (junction 42) [order 2] : [IDin!=ID2]
    (junction 63) -> (junction 66)
    (junction 42) -> (junction 66) [order 1] : [VTPM_WritingCnt_enum==2]
        | {ID4=IDin;....
        | ID4pressure=VINP_Pin_raw8;....
        | ID4Temp=VINP_Tin_raw8;}
  state GetID
    en:TPMSTLCmd=0;
  state LearnFail
    en:LProgress=3;
    state W1
      en:TPMSTLCmd=0;
    state W2
      en:TPMSTLCmd=1;
    state W3
      en:TPMSTLCmd=0;
    state W4
      en:TPMSTLCmd=1;
    (default) -> W1
    W1 -> W2 : [after(50,tick)]
    W2 -> W3 : [after(50,tick)]
    W3 -> W4 : [after(50,tick)]
  state Finish
    en:fDone=1;
    LProgress=1;
  (default) -> StandBy : {LProgress=0;}
  StandBy -> Learning : [DiagLearn]{VTPM_WritingCnt_enum=0;}
  GetID -> Learning : [after(100,tick)]
  Learning -> LearnFail : [after(6000,tick)]
  (junction 66) -> GetID : {VTPM_WritingCnt_enum=VTPM_WritingCnt_enum+1;}
  (junction 42) -> (junction 49) [order 2] : [IDin!=ID4]
      | {ID3=IDin;....
      | ID3pressure=VINP_Pin_raw8;....
      | ID3Temp=VINP_Tin_raw8;}
  W4 -> StandBy : [after(50,tick)]
  Finish -> StandBy
  (junction 49) -> Finish
  data: DataIn input; ID1 output uint32; ID2 output uint32; ID3 output uint32; ID4 output uint32; TPMSTLCmd output boolean; IDin input; DiagLearn input; fDone output boolean; VINP_Pin_raw8 input; VINP_Tin_raw8 input; ID1pressure output uint8; ID2pressure output uint8; ID3pressure output uint8; ID4pressure output uint8; ID1Temp output single; ID2Temp output single; ID3Temp output single; ID4Temp output single; VTPM_WritingCnt_enum output uint8; VINP_TPMSTrigger_flg input; LProgress output uint8

== stateflow chart tpm/TPM/TPMS/TPMS/Learn/LowerTirePressureCalibration/WarningPressureLearn3 ==
  state WarningPressureLearn [parallel]
    settings: executionOrder=1
    state Standby
      en:
      C=0;
      P=0;
      T=0;
      VTPM_P3alarm_raw=93;
      SPressindi=0;
    state Status
      en:
      P=P+VINP_Pin_raw8;
      T=T+VINP_Tin_raw8;
      C=C+1;
      SPressindi=3;
    state Calculate
      en:
      Pavg=P>>2;
      Tavg=T>>2;
      Pavg20=(Pavg*1.72+151)*(273+20)/(273+Tavg)-101;
    state Nopass
      en:
      SPressindi=2;
    state Pass
      en:
      SPressindi=1;
      VTPM_P3alarm_raw=(Pavg20*0.8+14-50)/1.72;
    (default) -> Standby
    Status -> Standby [order 2] : [VINP_TPMSResButt_flg||VINP_TPMSCaliButt_flg||VTPM_S3timeout_flg]
    Status -> Calculate [order 1] : [C>=4]
    Standby -> (junction 217) : [VINP_DATAin_flg&&!VINP_TPMSResButt_flg&&(VTPM_IDLOCK_flg||VTPM_LocationDone_flg)]
    (junction 217) -> Status : [VINP_IDin_raw32==VTPM_S3ID_raw32....
        | &&VINP_Pin_raw8!=0&&VINP_Tin_raw8!=0]
    (junction 235) -> (junction 217)
    Status -> (junction 235) [order 3] : [VINP_DATAin_flg&&C<4]
    (junction 69) -> Nopass [order 2]
    Calculate -> (junction 69)
    Nopass -> Standby : [VINP_TPMSResButt_flg||VINP_TPMSCaliButt_flg]
    (junction 69) -> Pass [order 1] : [Pavg20>245]
    Pass -> Standby : [VINP_TPMSResButt_flg||VINP_TPMSCaliButt_flg]
  data: VINP_Pin_raw8 input; VINP_Tin_raw8 input; VINP_IDin_raw32 input; VINP_DATAin_flg input; VINP_TPMSResButt_flg input; VINP_TPMSCaliButt_flg input; VTPM_IDLOCK_flg input; VTPM_P3alarm_raw output uint8; Pavg20 local single; SPressindi output uint8; P local single; Pavg local single; T local single; Tavg local single; VTPM_S3ID_raw32 input; C local uint8; VTPM_LocationDone_flg input; VTPM_S3timeout_flg input

== matlab function tpm/TPM/TPMS/TPMS/Learn/AutoLocation/IDIdentify/Subsystem7/Enabled Subsystem1/MATLAB Function ==
  data: C input; S output; Min input; X2 input; X3 input; X4 input; Y2 output; Y3 output; Y4 output; X5 input; X6 input; X7 input; X8 input; X9 input; Y5 output; Y6 output; Y7 output; Y8 output; Y9 output
function [S,Y2,Y3,Y4,Y5,Y6,Y7,Y8,Y9]   = fcn(C,Min,X2,X3,X4,X5,X6,X7,X8,X9)
Y=int16([X2 X3 X4 X5 X6 X7 X8 X9 Min]);
if (C<9)
    S=300;
else
    B=sort(Y);
    D=zeros(1,length(B));
    for i=1:1:length(D)
        if (i~=length(D))
            D(i)=B(i+1)-B(i);
        else
            if (B(length(D))-B(1)>B(1)+96-B(length(D)))
                D(length(D))=B(1)+96-B(length(D));
            else
                D(length(D))=B(length(D))-B(1);
            end
        end
    end

    [K,I]=sort(D);
    S=sum(K(1:7));
end
Y2=Y(2);
Y3=Y(3);
Y4=Y(4);
Y5=Y(5);
Y6=Y(6);
Y7=Y(7);
Y8=Y(8);
Y9=Y(9);

== stateflow chart tpm/TPM/TPMS/TPMS/Learn/LowerTirePressureCalibration/WarningPressureLearn4 ==
  state WarningPressureLearn [parallel]
    settings: executionOrder=1
    state Standby
      en:
      C=0;
      P=0;
      T=0;
      VTPM_P4alarm_raw=93;
      SPressindi=0;
    state Status
      en:
      P=P+VINP_Pin_raw8;
      T=T+VINP_Tin_raw8;
      C=C+1;
      SPressindi=3;
    state Calculate
      en:
      Pavg=P>>2;
      Tavg=T>>2;
      Pavg20=(Pavg*1.72+151)*(273+20)/(273+Tavg)-101;
    state Nopass
      en:
      SPressindi=2;
    state Pass
      en:
      SPressindi=1;
      VTPM_P4alarm_raw=(Pavg20*0.8+14-50)/1.72;
    (default) -> Standby
    Status -> Standby [order 2] : [VINP_TPMSResButt_flg||VINP_TPMSCaliButt_flg||VTPM_S4timeout_flg]
    Status -> Calculate [order 1] : [C>=4]
    Standby -> (junction 217) : [VINP_DATAin_flg&&!VINP_TPMSResButt_flg&&(VTPM_IDLOCK_flg||VTPM_LocationDone_flg)]
    (junction 217) -> Status : [VINP_IDin_raw32==VTPM_S4ID_raw32....
        | &&VINP_Pin_raw8!=0&&VINP_Tin_raw8!=0]
    (junction 235) -> (junction 217)
    Status -> (junction 235) [order 3] : [VINP_DATAin_flg&&C<4]
    (junction 69) -> Nopass [order 2]
    Calculate -> (junction 69)
    Nopass -> Standby : [VINP_TPMSResButt_flg||VINP_TPMSCaliButt_flg]
    (junction 69) -> Pass [order 1] : [Pavg20>245]
    Pass -> Standby : [VINP_TPMSResButt_flg||VINP_TPMSCaliButt_flg]
  data: VINP_Pin_raw8 input; VINP_Tin_raw8 input; VINP_IDin_raw32 input; VINP_DATAin_flg input; VINP_TPMSResButt_flg input; VINP_TPMSCaliButt_flg input; VTPM_IDLOCK_flg input; VTPM_P4alarm_raw output uint8; Pavg20 local single; SPressindi output uint8; P local single; Pavg local single; T local single; Tavg local single; VTPM_S4ID_raw32 input; C local uint8; VTPM_LocationDone_flg input; VTPM_S4timeout_flg input

== stateflow chart tpm/TPM/TPMS/TPMS/Learn/AutoLocation/IDIdentify/Subsystem2/Chart1 ==
  state GCal [parallel]
    settings: executionOrder=1
    state NoSignal
      en:G=false;
    state SignalIn
      en:G=true;
    (default) -> NoSignal
    NoSignal -> (junction 17) : [VINP_DATAin_flg]
    (junction 17) -> SignalIn [order 1] : [!Used]
    (junction 17) -> (junction 19) [order 2]
    (junction 19) -> NoSignal [order 2]
    (junction 19) -> SignalIn [order 1] : [VINP_IDin_raw32==IDout]
    SignalIn -> NoSignal
  state timecounter [parallel]
    settings: executionOrder=3
    state standby
      en:
      VTPM_S3timeout_flg=0;
      VTPM_timeout_cnt=0;
    state counter
      during:
      VTPM_timeout_cnt=VTPM_timeout_cnt+1;
    state stopcounter
    state timeout
      en:
      VTPM_S3timeout_flg=1;
    (default) -> standby
    (junction 68) -> standby
    (junction 63) -> (junction 68)
    standby -> counter : [Used&&!VTPM_FlashIDlock_flg]
    counter -> standby [order 1] : [!Used||(VINP_DATAin_flg&&IDout==VINP_IDin_raw32)]
    stopcounter -> counter : [VINP_VehSpeed_kph>=KTPM_DataInVehSpdThreshold_kph]
    counter -> stopcounter [order 3] : [VINP_VehSpeed_kph<KTPM_DataInVehSpdThreshold_kph]
    counter -> timeout [order 2] : [VTPM_timeout_cnt>12000]
    timeout -> (junction 63)
  state IDCheck [parallel]
    settings: executionOrder=2
    state FlashID
      en:
      IDout=VINP_S3ID_raw;
      Used=true;
      VTPM_S3IDLock_flg=true;
    state Unused
      en:IDout=0;
      VTPM_S3IDLock_flg=false;
      Used=false;
      IDLock_cnt=0;
    state VINP_DATAin_flg
      state Used
        en:IDout=VINP_IDin_raw32;
        Used=true;
        IDLock_cnt=IDLock_cnt+1;
      state Lock
        en:VTPM_S3IDLock_flg=true;
      Used -> Used [order 2] : [VINP_DATAin_flg&&IDout==VINP_IDin_raw32]
      Used -> Lock [order 1] : [IDLock_cnt>=4]
    (default) -> Unused
    Unused -> FlashID [order 1] : [VTPM_FlashIDlock_flg||VTPM_TPMSmanualDone_flg]
    FlashID -> Unused : [VINP_TPMSResButt_flg]
    Unused -> Used [order 2] : [VINP_DATAin_flg]
    Used -> Unused [order 3] : [VTPM_S3timeout_flg==1]
    VINP_DATAin_flg -> FlashID [order 2] : [VTPM_TPMSmanualDone_flg]
    VINP_DATAin_flg -> Unused [order 1] : [VINP_TPMSResButt_flg]
  data: VINP_IDin_raw32 input; VINP_TPMSResButt_flg input; VINP_DATAin_flg input; G output boolean; Used output boolean; VTPM_S3IDLock_flg output boolean; IDout output uint32; VTPM_FlashIDlock_flg input; VINP_S3ID_raw input; VINP_VehSpeed_kph input; IDLock_cnt local uint32; VTPM_timeout_cnt local uint32; VTPM_S3timeout_flg output boolean; VTPM_TPMSmanualDone_flg input; KTPM_DataInVehSpdThreshold_kph input

== matlab function tpm/TPM/TPMS/TPMS/Learn/AutoLocation/IDIdentify/Subsystem7/Enabled Subsystem2/MATLAB Function ==
  data: C input; S output; Min input; X2 input; X3 input; X4 input; Y2 output; Y3 output; Y4 output; X5 input; X6 input; X7 input; X8 input; X9 input; Y5 output; Y6 output; Y7 output; Y8 output; Y9 output
function [S,Y2,Y3,Y4,Y5,Y6,Y7,Y8,Y9]   = fcn(C,Min,X2,X3,X4,X5,X6,X7,X8,X9)
Y=int16([X2 X3 X4 X5 X6 X7 X8 X9 Min]);
if (C<9)
    S=300;
else
    B=sort(Y);
    D=zeros(1,length(B));
    for i=1:1:length(D)
        if (i~=length(D))
            D(i)=B(i+1)-B(i);
        else
            if (B(length(D))-B(1)>B(1)+96-B(length(D)))
                D(length(D))=B(1)+96-B(length(D));
            else
                D(length(D))=B(length(D))-B(1);
            end
        end
    end

    [K,I]=sort(D);
    S=sum(K(1:7));
end
Y2=Y(2);
Y3=Y(3);
Y4=Y(4);
Y5=Y(5);
Y6=Y(6);
Y7=Y(7);
Y8=Y(8);
Y9=Y(9);

== stateflow chart tpm/TPM/TPMS/TPMS/Learn/AutoLocation/WheelPosition/Chart3 ==
  state Start
    state Forward
      en:
      a=(VTPM_LRWpos_raw+Delta);
      b=(VTPM_LRWpos_raw+Delta)/96;
      VTPM_LRWpos_raw=a-b*96;
    state Else
    state Backward
      en:
      a=(VTPM_LRWpos_raw+Delta);
      b=(VTPM_LRWpos_raw+Delta)/96;
      VTPM_LRWpos_raw=a-b*96;
    (default) -> (junction 54) : {VTPM_LRWpos_raw=0; Delta=0; PulseCountBuf=VINP_LRPulseCount_cnt;}
    Start -> (junction 54) : [hasChanged(VINP_LRPulseCount_cnt)]....
        | {Delta=VINP_LRPulseCount_cnt-PulseCountBuf;
        | PulseCountBuf=VINP_LRPulseCount_cnt;}
    (junction 54) -> (junction 47) [order 1] : [VPMM_PowerSta_enum!=ENUM_PWRSTASW_OFF&&....
        |  VPMM_PowerSta_enum!=ENUM_PWRSTASW_OFFCHVCHRG&&...
        |  VPMM_PowerSta_enum!=ENUM_PWRSTASW_OFFA&&....
        |  VPMM_PowerSta_enum!=ENUM_PWRSTASW_STANDBY&&....
        |  VINP_LRPulseCountV_flg==false]
    (junction 47) -> (junction 6) [order 1] : [VTPM_LRWhlRotDir_enum==1]
    (junction 6) -> Forward [order 1] : [Delta>0]
    (junction 54) -> Else [order 2]
    (junction 47) -> (junction 48) [order 2]
    (junction 6) -> (junction 10) [order 2] : [Delta<0]
    (junction 10) -> Forward : {Delta=Delta+256;}
    (junction 48) -> Else [order 2]
    (junction 48) -> (junction 14) [order 1] : [VTPM_LRWhlRotDir_enum==2]
    (junction 14) -> Backward [order 1] : [Delta>0]{Delta=-Delta+96;}
    (junction 14) -> (junction 16) [order 2] : [Delta<0]
    (junction 16) -> Backward : {Delta=-Delta+128;}
  data: VPMM_PowerSta_enum input; VINP_LRPulseCount_cnt input; VINP_LRPulseCountV_flg input; VTPM_LRWhlRotDir_enum input; VTPM_LRWpos_raw output int16; a local int16; b local int16; Delta local int16; PulseCountBuf local int16; ENUM_PWRSTASW_OFF parameter; ENUM_PWRSTASW_OFFA parameter; ENUM_PWRSTASW_OFFCHVCHRG parameter; ENUM_PWRSTASW_STANDBY parameter

== matlab function tpm/TPM/TPMS/TPMS/Learn/AutoLocation/IDIdentify/Enabled Subsystem/MATLAB Function ==
  data: VINP_TPMSResButt_flg input; S1L output; VTPM_LFS1_cnt input; VTPM_RFS1_cnt input; VTPM_LRS1_cnt input; VTPM_RRS1_cnt input; VTPM_LFS2_cnt input; VTPM_RFS2_cnt input; VTPM_LRS2_cnt input; VTPM_RRS2_cnt input; VTPM_LFS3_cnt input; VTPM_RFS3_cnt input; VTPM_LRS3_cnt input; VTPM_RRS3_cnt input; VTPM_LFS4_cnt input; VTPM_RFS4_cnt input; VTPM_LRS4_cnt input; VTPM_RRS4_cnt input; S2L output; S3L output; S4L output
 function [S1L,S2L,S3L,S4L] = fcn(VINP_TPMSResButt_flg,VTPM_LFS1_cnt,VTPM_RFS1_cnt,VTPM_LRS1_cnt,VTPM_RRS1_cnt,VTPM_LFS2_cnt,VTPM_RFS2_cnt,VTPM_LRS2_cnt,VTPM_RRS2_cnt,VTPM_LFS3_cnt,VTPM_RFS3_cnt,VTPM_LRS3_cnt,VTPM_RRS3_cnt,VTPM_LFS4_cnt,VTPM_RFS4_cnt,VTPM_LRS4_cnt,VTPM_RRS4_cnt)

if (VINP_TPMSResButt_flg)
    S1L=0;
    S2L=0;
    S3L=0;
    S4L=0;
else
    SL=zeros(1,4);
    S1S=[VTPM_LFS1_cnt VTPM_RFS1_cnt VTPM_LRS1_cnt VTPM_RRS1_cnt];
    S2S=[VTPM_LFS2_cnt VTPM_RFS2_cnt VTPM_LRS2_cnt VTPM_RRS2_cnt];
    S3S=[VTPM_LFS3_cnt VTPM_RFS3_cnt VTPM_LRS3_cnt VTPM_RRS3_cnt];
    S4S=[VTPM_LFS4_cnt VTPM_RFS4_cnt VTPM_LRS4_cnt VTPM_RRS4_cnt];
    S=[S1S;S2S;S3S;S4S];
 for i=1:4
    [AS1,AS1I]=sort(S(1,:));
    [AS2,AS2I]=sort(S(2,:));
    [AS3,AS3I]=sort(S(3,:));
    [AS4,AS4I]=sort(S(4,:));
    DifA=[AS1(2)-AS1(1) AS2(2)-AS2(1) AS3(2)-AS3(1) AS4(2)-AS4(1)];
    [DifASort,DifAI]=sort(DifA);
    [BS1,BS1I]=sort(S(:,1));
    [BS2,BS2I]=sort(S(:,2));
    [BS3,BS3I]=sort(S(:,3));
    [BS4,BS4I]=sort(S(:,4));
    DifB=[BS1(2)-BS1(1) BS2(2)-BS2(1) BS3(2)-BS3(1) BS4(2)-BS4(1)];
    [DifBSort,DifBI]=sort(DifB);
    if (DifASort(4)>DifBSort(4))
        S(DifAI(4),:)=ones(1,4)*255;
        if DifAI(4)==1
            SL(DifAI(4))=AS1I(1);
            S(:,AS1I(1))=ones(4,1)*255;
        elseif DifAI(4)==2
            SL(DifAI(4))=AS2I(1);
            S(:,AS2I(1))=ones(4,1)*255;
        elseif DifAI(4)==3
            SL(DifAI(4))=AS3I(1);
            S(:,AS3I(1))=ones(4,1)*255;
        else
            SL(DifAI(4))=AS4I(1);
            S(:,AS4I(1))=ones(4,1)*255;
        end
    else
        S(:,DifBI(4))=ones(4,1)*255;
        if DifBI(4)==1
            SL(BS1I(1))=DifBI(4);
            S(BS1I(1),:)=ones(1,4)*255;
        elseif DifBI(4)==2
            SL(BS2I(1))=DifBI(4);
            S(BS2I(1),:)=ones(1,4)*255;
        elseif DifBI(4)==3
            SL(BS3I(1))=DifBI(4);
            S(BS3I(1),:)=ones(1,4)*255;
        else
            SL(BS4I(1))=DifBI(4);
            S(BS4I(1),:)=ones(1,4)*255;
        end
    end
end

    S1L=SL(1);
    S2L=SL(2);
    S3L=SL(3);
    S4L=SL(4);
end

== matlab function tpm/TPM/TPMS/TPMS/Learn/AutoLocation/IDIdentify/Subsystem7/Enabled Subsystem3/MATLAB Function ==
  data: C input; S output; Min input; X2 input; X3 input; X4 input; Y2 output; Y3 output; Y4 output; X5 input; X6 input; X7 input; X8 input; X9 input; Y5 output; Y6 output; Y7 output; Y8 output; Y9 output
function [S,Y2,Y3,Y4,Y5,Y6,Y7,Y8,Y9]   = fcn(C,Min,X2,X3,X4,X5,X6,X7,X8,X9)
Y=int16([X2 X3 X4 X5 X6 X7 X8 X9 Min]);
if (C<9)
    S=300;
else
    B=sort(Y);
    D=zeros(1,length(B));
    for i=1:1:length(D)
        if (i~=length(D))
            D(i)=B(i+1)-B(i);
        else
            if (B(length(D))-B(1)>B(1)+96-B(length(D)))
                D(length(D))=B(1)+96-B(length(D));
            else
                D(length(D))=B(length(D))-B(1);
            end
        end
    end

    [K,I]=sort(D);
    S=sum(K(1:7));
end
Y2=Y(2);
Y3=Y(3);
Y4=Y(4);
Y5=Y(5);
Y6=Y(6);
Y7=Y(7);
Y8=Y(8);
Y9=Y(9);
